simulink model "Motor_rotate_simulation1"  (R2017b)
settings: Solver=VariableStepAuto  StartTime=0.0  StopTime=10  RelTol=1e-3
values from neighbouring files (symbols this model uses):
  PPR = 10000    [matlab.mat]
  T = 0.02    [matlab.mat]
libraries: arduino_io_lib x4
settings Model: Creator=MrGoshak  LastModifiedBy=MrGoshak

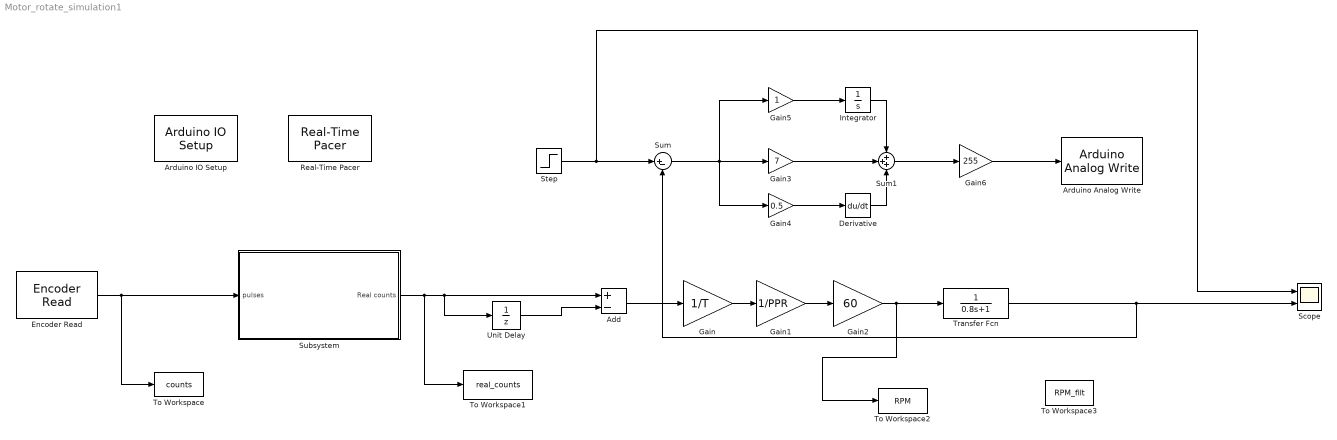
== system Motor_rotate_simulation1 ==
  Add : Sum  Inputs=+-
  Arduino Analog Write : arduino_io_lib/Arduino Analog Write  arduinoVar=Temporary arduino variable: Arduino1  arduinoPin=5  T=0.06
  Arduino IO Setup : arduino_io_lib/Arduino IO Setup  Priority=3  arduinoVar=Temporary arduino variable: Arduino1  workspaceVarName=a  comPort=COM3
  Derivative : Derivative
  Encoder Read : arduino_io_lib/Encoder Read  arduinoVar=Temporary arduino variable: Arduino1  encNum=1  pinA=2  pinB=3  DbDl=0  T=T
  Gain : Gain  Gain=1/T
  Gain1 : Gain  Gain=1/PPR
  Gain2 : Gain  Gain=60
  Gain3 : Gain  Gain=7
  Gain4 : Gain  Gain=0.5
  Gain5 : Gain
  Gain6 : Gain  Gain=255
  Integrator : Integrator
  Real-Time Pacer : arduino_io_lib/Real-Time Pacer  simTimePerRealTime=1
  Scope : Scope  NumInputPorts=2
  Step : Step  After=16  SampleTime=T
  Subsystem : Subsystem
  Sum : Sum  Inputs=|+-
  Sum1 : Sum  Inputs=+++
  To Workspace : ToWorkspace  VariableName=counts  SaveFormat=Timeseries  SampleTime=-1
  To Workspace1 : ToWorkspace  VariableName=real_counts  SaveFormat=Timeseries  SampleTime=-1
  To Workspace2 : ToWorkspace  VariableName=RPM  SaveFormat=Timeseries  SampleTime=-1
  To Workspace3 : ToWorkspace  VariableName=RPM_filt  SampleTime=-1
      settings: Save2DSignal=2-D array (concatenate along first dimension)
  Transfer Fcn : TransferFcn  Denominator=[0.8 1]
  Unit Delay : UnitDelay  SampleTime=T
  wires:
  Encoder Read/1 -> Subsystem/1(pulses), To Workspace/1
  Subsystem/1(Real counts) -> Unit Delay/1, Add/1, To Workspace1/1
  Unit Delay/1 -> Add/2
  Add/1 -> Gain/1
  Gain/1 -> Gain1/1
  Gain1/1 -> Gain2/1
  Gain2/1 -> Transfer Fcn/1, To Workspace2/1
  Step/1 -> Scope/1, Sum/1
  Integrator/1 -> Sum1/1
  Derivative/1 -> Sum1/3
  Gain5/1 -> Integrator/1
  Gain4/1 -> Derivative/1
  Gain3/1 -> Sum1/2
  Gain6/1 -> Arduino Analog Write/1
  Transfer Fcn/1 -> Sum/2, Scope/2
  Sum/1 -> Gain3/1, Gain4/1, Gain5/1
  Sum1/1 -> Gain6/1

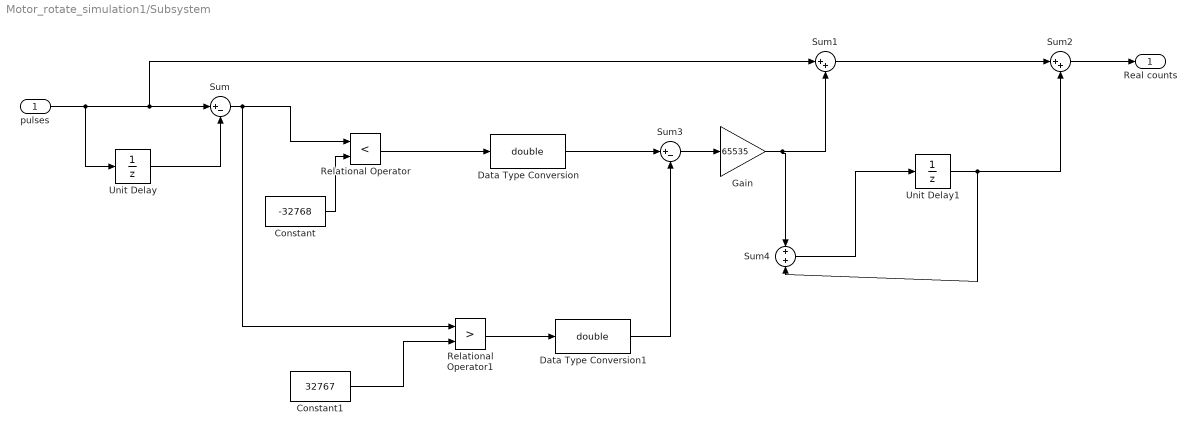
== system Motor_rotate_simulation1/Subsystem ==
  pulses : Inport
  Constant : Constant  Value=-32768  VectorParams1D=off
  Constant1 : Constant  Value=32767  VectorParams1D=off
  Data Type Conversion : DataTypeConversion  OutDataTypeStr=double
  Data Type Conversion1 : DataTypeConversion  OutDataTypeStr=double
  Gain : Gain  Gain=65535
  Relational Operator : RelationalOperator  Operator=<  OutDataTypeStr=boolean  RndMeth=Simplest
  Relational Operator1 : RelationalOperator  Operator=>  OutDataTypeStr=boolean  RndMeth=Simplest
  Sum : Sum  Inputs=|+-
  Sum1 : Sum  Inputs=|++
  Sum2 : Sum  Inputs=|++
  Sum3 : Sum  Inputs=|+-
  Sum4 : Sum
  Unit Delay : UnitDelay  SampleTime=-1
  Unit Delay1 : UnitDelay  SampleTime=-1
  Real counts : Outport
  wires:
  Sum/1 -> Relational Operator1/1, Relational Operator/1
  Constant/1 -> Relational Operator/2
  Sum1/1 -> Sum2/1
  pulses/1 -> Unit Delay/1, Sum1/1, Sum/1
  Unit Delay/1 -> Sum/2
  Constant1/1 -> Relational Operator1/2
  Sum2/1 -> Real counts/1
  Gain/1 -> Sum4/1, Sum1/2
  Sum4/1 -> Unit Delay1/1
  Unit Delay1/1 -> Sum4/2, Sum2/2
  Data Type Conversion/1 -> Sum3/1
  Sum3/1 -> Gain/1
  Relational Operator1/1 -> Data Type Conversion1/1
  Data Type Conversion1/1 -> Sum3/2
  Relational Operator/1 -> Data Type Conversion/1
